simulink model "old_CascadePID_sim_v1"  (R2024b)
settings: Solver=ode4  StartTime=0.0  StopTime=30  FixedStep=0.05  RelTol=1e-3
values from neighbouring files (symbols this model uses):
  b_moment = 5.4e-6    (= 5.4e-06)    [CascadePID_matlab_client_v1.m]    (also in old_CascadePID_matlab_client_v1.m)
  k_thrust = 2.3e-3    (= 0.0023)    [CascadePID_matlab_client_v1.m]    (also in old_CascadePID_matlab_client_v1.m)
  l = 0.2051    [CascadePID_matlab_client_v1.m]    (also in old_CascadePID_matlab_client_v1.m)
libraries: slpidlib x9, simulink_extras x7
settings Model: Creator=Admin  LastModifiedBy=Admin

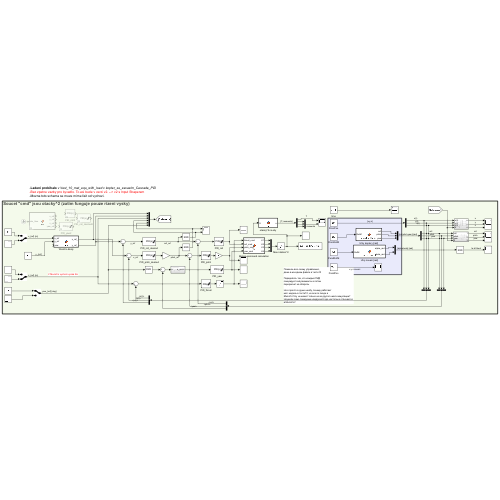
[thumbnail: Simulink's stored preview of the top-level diagram]
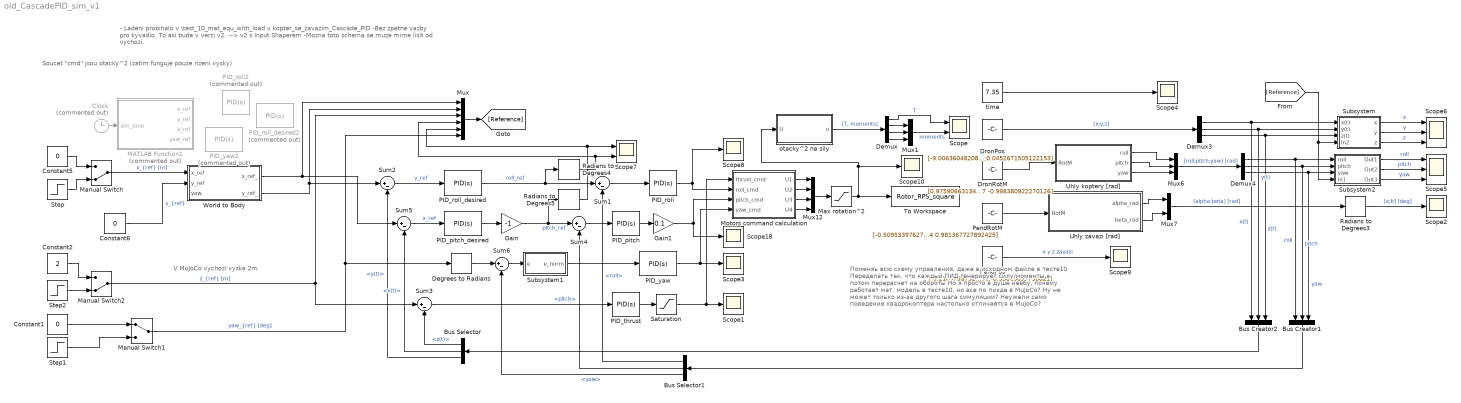
== system old_CascadePID_sim_v1 ==
  note: Поменяь всю схему управления,
      | даже в исходном файле в тесте10
      |
      | Переделать так, что каждый ПИД
      | генерирует силу/моменты а потом
      | перерасчет на обороты
      |
      | Но я просто в душе неебу, почему работает
      | мат. модель в тесте10, но все по пизде в
      | MuJoCo? Ну не может только из-за другого шага симуляции?
      | Неужели само поведение квадрокоптера настолько отличается
      | в MuJoCo?
  note: V MuJoCo vychozi vyska 2m
  note: - Ladeni probihalo v \test_10_mat_equ_with_load v kopter_se_zavazim_Cascade_PID
      | -Bez zpetne vazby pro kyvadlo. To asi bude v verzi v2. --> v2 s Input Shaperem
      | -Mozna toto schema se muze mirne lisit od vychozi.
  note: Soucet "cmd" jsou otacky^2 (zatim funguje pouze rizeni vysky)
  Bus Creator1 : BusCreator  Inputs=3
  Bus Creator2 : BusCreator  Inputs=3
  Bus Selector : BusSelector  OutputSignals=z(t),x(t),y(t)
  Bus Selector1 : BusSelector  OutputSignals=roll,pitch,yaw
  Clock : Clock  Commented=on
  Constant1 : Constant  Value=0
  Constant2 : Constant  Value=2
  Constant5 : Constant  Value=0
  Constant6 : Constant  Value=0
  Degrees to Radians : simulink_extras/Transformations/Degrees to Radians
  Demux : Demux
  Demux3 : Demux  Outputs=3
  Demux4 : Demux  Outputs=3
  DronPos : Constant  Value=[-9.00636048208464;0.341459514164713;0.0452671505122153]  SampleTime=-1
  DronRotM : Constant  Value=[0.975906631347119 0.216434408196844 -0.0276114802428831;0.214907774343092 -0.975367370953657 -0.0497306767081764;-0.0376947664752024 0.0425985754155727 -0.998380922270126]  SampleTime=-1
  Gain : Gain  Gain=-1
  Gain1 : Gain  Gain=0.1
  MATLAB Function1 : MATLAB Function  Commented=on  TreatAsAtomicUnit=on
  Manual Switch : ManualSwitch  CurrentSetting=0
  Manual Switch1 : ManualSwitch
  Manual Switch2 : ManualSwitch  CurrentSetting=0
  Max rotation^2 : Saturate  UpperLimit=4200  LowerLimit=0  LinearizeAsGain=off
  Motors command calculation : MATLAB Function  TreatAsAtomicUnit=on
  Mux : Mux  Inputs=6
  Mux1 : Mux  Inputs=3
  Mux12 : Mux
  Mux6 : Mux  Inputs=3
  Mux7 : Mux  Inputs=2
  PID_pitch : slpidlib/PID Controller  Controller=PID  Form=Parallel  TimeDomain=Continuous-time  UseExternalTs=off  SampleTime=-1  IntegratorMethod=Forward Euler  FilterMethod=Forward Euler  ControllerParametersSource=internal  P=218.455453578619  I=102.269436232904  UseKiTs=off  D=114.583796831467  UseExternalDerivativeSource=off  N=54.5397025421619  UseFilter=on  TunerSelectOption=Transfer Function Based (PID Tuner App)  InitialConditionSource=internal  InitialConditionForIntegrator=0  InitialConditionForFilter=0  DifferentiatorICPrevScaledInput=0  ExternalReset=none  TrackingMode=off  Kt=1  LimitOutput=on  SatLimitsSource=internal  UpperSaturationLimit=500  LowerSaturationLimit=-500  LinearizeAsGain=off  AntiWindupMode=clamping  Kb=1  LimitIntegrator=off  UpperIntegratorSaturationLimit=inf  LowerIntegratorSaturationLimit=-inf  POutMin=[]  POutMax=[]  IOutMin=[]  IOutMax=[]  DOutMin=[]  DOutMax=[]  NOutMin=[]  NOutMax=[]  SumOutMin=[]  SumOutMax=[]  SaturationOutMin=[]  SaturationOutMax=[]  PParamMin=[]  PParamMax=[]  IParamMin=[]  IParamMax=[]  DParamMin=[]  DParamMax=[]  NParamMin=[]  NParamMax=[]  KbParamMin=[]  KbParamMax=[]  KtParamMin=[]  KtParamMax=[]  KbOutMin=[]  KbOutMax=[]  KtOutMin=[]  KtOutMax=[]  IntegratorOutMin=[]  IntegratorOutMax=[]  FilterOutMin=[]  FilterOutMax=[]  SumI1OutMin=[]  SumI1OutMax=[]  SumI2OutMin=[]  SumI2OutMax=[]  SumI3OutMin=[]  SumI3OutMax=[]  SumI4OutMin=[]  SumI4OutMax=[]  SumDOutMin=[]  SumDOutMax=[]  DifferentiatorOutMin=[]  DifferentiatorOutMax=[]  FilterDiffOutCoefMin=[]  FilterDiffOutCoefMax=[]  ReciprocalOutMin=[]  ReciprocalOutMax=[]  SumDenOutMin=[]  SumDenOutMax=[]  SumNumOutMin=[]  SumNumOutMax=[]  DivideOutMin=[]  DivideOutMax=[]  UdiffTsProdOutMin=[]  UdiffTsProdOutMax=[]  NTsProdOutMin=[]  NTsProdOutMax=[]  UintegralTsProdOutMin=[]  UintegralTsProdOutMax=[]  UngainTsProdOutMin=[]  UngainTsProdOutMax=[]  ClampingZeroOutDataTypeStr=Inherit: Inherit via back propagation  ClampingZeroOutMin=[]  ClampingZeroOutMax=[]  FilterDenConstantOutDataTypeStr=Inherit: Inherit via back propagation  FilterDenConstantOutMin=[]  FilterDenConstantOutMax=[]  PCopyOutDataTypeStr=Inherit: Inherit via back propagation  PCopyOutMin=[]  PCopyOutMax=[]  NCopyOutDataTypeStr=Inherit: Inherit via back propagation  NCopyOutMin=[]  NCopyOutMax=[]  IntegratorContinuousStateAttributes=''  IntegratorStateMustResolveToSignalObject=off  IntegratorRTWStateStorageClass=Auto  FilterContinuousStateAttributes=''  FilterStateMustResolveToSignalObject=off  FilterRTWStateStorageClass=Auto  ParallelPVariant=InternalParameters  IdealPVariant=Disabled  IVariant=InternalParameters  DVariant=InternalParameters  IntegratorVariant=Continuous  SatVariant=Enabled  AWVariant=ContClampingParallel  PCopyVariant=Disabled  TRVariant=Disabled  FdbkBlocksVariant=Forward  IdealPFdbkVariant=Disabled  SatFdbkVariant=Disabled  DerivativeFilterVariant=ContFilter  NVariant=InternalParameters  NCopyVariant=Disabled  FilterICVariant=InternalICsFilter  IntegratorICVariant=InternalICs  ExternalResetVariant=Disabled  TRSumVariant=Passthrough  SumFdbkVariant=Disabled  SumVariant=Sum_PID  TsampFilterVariant=InternalTs  TsampNgainVariant=Passthrough  TsampIntegralVariant=Disabled_SignalSpec  ExternalSaturationOutDataTypeStr=Inherit: Same as second input  DerivativeSourceVariant=ErrorSignal  PreIntVariant=InternalPreInt
  PID_pitch_desired : slpidlib/PID Controller  Controller=PID  Form=Parallel  TimeDomain=Continuous-time  UseExternalTs=off  SampleTime=-1  IntegratorMethod=Forward Euler  FilterMethod=Forward Euler  ControllerParametersSource=internal  P=-0.0958604126455568  I=-0.00355407713511052  UseKiTs=off  D=-0.176236133491369  UseExternalDerivativeSource=off  N=18.7292151918558  UseFilter=on  TunerSelectOption=Transfer Function Based (PID Tuner App)  InitialConditionSource=internal  InitialConditionForIntegrator=0  InitialConditionForFilter=0  DifferentiatorICPrevScaledInput=0  ExternalReset=none  TrackingMode=off  Kt=1  LimitOutput=on  SatLimitsSource=internal  UpperSaturationLimit=45*pi/180  LowerSaturationLimit=-45*pi/180  LinearizeAsGain=on  AntiWindupMode=clamping  Kb=1  LimitIntegrator=off  UpperIntegratorSaturationLimit=inf  LowerIntegratorSaturationLimit=-inf  POutMin=[]  POutMax=[]  IOutMin=[]  IOutMax=[]  DOutMin=[]  DOutMax=[]  NOutMin=[]  NOutMax=[]  SumOutMin=[]  SumOutMax=[]  SaturationOutMin=[]  SaturationOutMax=[]  PParamMin=[]  PParamMax=[]  IParamMin=[]  IParamMax=[]  DParamMin=[]  DParamMax=[]  NParamMin=[]  NParamMax=[]  KbParamMin=[]  KbParamMax=[]  KtParamMin=[]  KtParamMax=[]  KbOutMin=[]  KbOutMax=[]  KtOutMin=[]  KtOutMax=[]  IntegratorOutMin=[]  IntegratorOutMax=[]  FilterOutMin=[]  FilterOutMax=[]  SumI1OutMin=[]  SumI1OutMax=[]  SumI2OutMin=[]  SumI2OutMax=[]  SumI3OutMin=[]  SumI3OutMax=[]  SumI4OutMin=[]  SumI4OutMax=[]  SumDOutMin=[]  SumDOutMax=[]  DifferentiatorOutMin=[]  DifferentiatorOutMax=[]  FilterDiffOutCoefMin=[]  FilterDiffOutCoefMax=[]  ReciprocalOutMin=[]  ReciprocalOutMax=[]  SumDenOutMin=[]  SumDenOutMax=[]  SumNumOutMin=[]  SumNumOutMax=[]  DivideOutMin=[]  DivideOutMax=[]  UdiffTsProdOutMin=[]  UdiffTsProdOutMax=[]  NTsProdOutMin=[]  NTsProdOutMax=[]  UintegralTsProdOutMin=[]  UintegralTsProdOutMax=[]  UngainTsProdOutMin=[]  UngainTsProdOutMax=[]  ClampingZeroOutDataTypeStr=Inherit: Inherit via back propagation  ClampingZeroOutMin=[]  ClampingZeroOutMax=[]  FilterDenConstantOutDataTypeStr=Inherit: Inherit via back propagation  FilterDenConstantOutMin=[]  FilterDenConstantOutMax=[]  PCopyOutDataTypeStr=Inherit: Inherit via back propagation  PCopyOutMin=[]  PCopyOutMax=[]  NCopyOutDataTypeStr=Inherit: Inherit via back propagation  NCopyOutMin=[]  NCopyOutMax=[]  IntegratorContinuousStateAttributes=''  IntegratorStateMustResolveToSignalObject=off  IntegratorRTWStateStorageClass=Auto  FilterContinuousStateAttributes=''  FilterStateMustResolveToSignalObject=off  FilterRTWStateStorageClass=Auto  ParallelPVariant=InternalParameters  IdealPVariant=Disabled  IVariant=InternalParameters  DVariant=InternalParameters  IntegratorVariant=Continuous  SatVariant=Enabled  AWVariant=ContClampingParallel  PCopyVariant=Disabled  TRVariant=Disabled  FdbkBlocksVariant=Forward  IdealPFdbkVariant=Disabled  SatFdbkVariant=Disabled  DerivativeFilterVariant=ContFilter  NVariant=InternalParameters  NCopyVariant=Disabled  FilterICVariant=InternalICsFilter  IntegratorICVariant=InternalICs  ExternalResetVariant=Disabled  TRSumVariant=Passthrough  SumFdbkVariant=Disabled  SumVariant=Sum_PID  TsampFilterVariant=InternalTs  TsampNgainVariant=Passthrough  TsampIntegralVariant=Disabled_SignalSpec  ExternalSaturationOutDataTypeStr=Inherit: Same as second input  DerivativeSourceVariant=ErrorSignal  PreIntVariant=InternalPreInt
  PID_roll : slpidlib/PID Controller  Controller=PID  Form=Parallel  TimeDomain=Continuous-time  UseExternalTs=off  SampleTime=-1  IntegratorMethod=Forward Euler  FilterMethod=Forward Euler  ControllerParametersSource=internal  P=218.455453578619  I=102.269436232904  UseKiTs=off  D=114.583796831467  UseExternalDerivativeSource=off  N=54.5397025421619  UseFilter=on  TunerSelectOption=Transfer Function Based (PID Tuner App)  InitialConditionSource=internal  InitialConditionForIntegrator=0  InitialConditionForFilter=0  DifferentiatorICPrevScaledInput=0  ExternalReset=none  TrackingMode=off  Kt=1  LimitOutput=on  SatLimitsSource=internal  UpperSaturationLimit=500  LowerSaturationLimit=-500  LinearizeAsGain=off  AntiWindupMode=clamping  Kb=1  LimitIntegrator=off  UpperIntegratorSaturationLimit=inf  LowerIntegratorSaturationLimit=-inf  POutMin=[]  POutMax=[]  IOutMin=[]  IOutMax=[]  DOutMin=[]  DOutMax=[]  NOutMin=[]  NOutMax=[]  SumOutMin=[]  SumOutMax=[]  SaturationOutMin=[]  SaturationOutMax=[]  PParamMin=[]  PParamMax=[]  IParamMin=[]  IParamMax=[]  DParamMin=[]  DParamMax=[]  NParamMin=[]  NParamMax=[]  KbParamMin=[]  KbParamMax=[]  KtParamMin=[]  KtParamMax=[]  KbOutMin=[]  KbOutMax=[]  KtOutMin=[]  KtOutMax=[]  IntegratorOutMin=[]  IntegratorOutMax=[]  FilterOutMin=[]  FilterOutMax=[]  SumI1OutMin=[]  SumI1OutMax=[]  SumI2OutMin=[]  SumI2OutMax=[]  SumI3OutMin=[]  SumI3OutMax=[]  SumI4OutMin=[]  SumI4OutMax=[]  SumDOutMin=[]  SumDOutMax=[]  DifferentiatorOutMin=[]  DifferentiatorOutMax=[]  FilterDiffOutCoefMin=[]  FilterDiffOutCoefMax=[]  ReciprocalOutMin=[]  ReciprocalOutMax=[]  SumDenOutMin=[]  SumDenOutMax=[]  SumNumOutMin=[]  SumNumOutMax=[]  DivideOutMin=[]  DivideOutMax=[]  UdiffTsProdOutMin=[]  UdiffTsProdOutMax=[]  NTsProdOutMin=[]  NTsProdOutMax=[]  UintegralTsProdOutMin=[]  UintegralTsProdOutMax=[]  UngainTsProdOutMin=[]  UngainTsProdOutMax=[]  ClampingZeroOutDataTypeStr=Inherit: Inherit via back propagation  ClampingZeroOutMin=[]  ClampingZeroOutMax=[]  FilterDenConstantOutDataTypeStr=Inherit: Inherit via back propagation  FilterDenConstantOutMin=[]  FilterDenConstantOutMax=[]  PCopyOutDataTypeStr=Inherit: Inherit via back propagation  PCopyOutMin=[]  PCopyOutMax=[]  NCopyOutDataTypeStr=Inherit: Inherit via back propagation  NCopyOutMin=[]  NCopyOutMax=[]  IntegratorContinuousStateAttributes=''  IntegratorStateMustResolveToSignalObject=off  IntegratorRTWStateStorageClass=Auto  FilterContinuousStateAttributes=''  FilterStateMustResolveToSignalObject=off  FilterRTWStateStorageClass=Auto  ParallelPVariant=InternalParameters  IdealPVariant=Disabled  IVariant=InternalParameters  DVariant=InternalParameters  IntegratorVariant=Continuous  SatVariant=Enabled  AWVariant=ContClampingParallel  PCopyVariant=Disabled  TRVariant=Disabled  FdbkBlocksVariant=Forward  IdealPFdbkVariant=Disabled  SatFdbkVariant=Disabled  DerivativeFilterVariant=ContFilter  NVariant=InternalParameters  NCopyVariant=Disabled  FilterICVariant=InternalICsFilter  IntegratorICVariant=InternalICs  ExternalResetVariant=Disabled  TRSumVariant=Passthrough  SumFdbkVariant=Disabled  SumVariant=Sum_PID  TsampFilterVariant=InternalTs  TsampNgainVariant=Passthrough  TsampIntegralVariant=Disabled_SignalSpec  ExternalSaturationOutDataTypeStr=Inherit: Same as second input  DerivativeSourceVariant=ErrorSignal  PreIntVariant=InternalPreInt
  PID_roll2 : slpidlib/PID Controller  Commented=on  Controller=PID  Form=Parallel  TimeDomain=Continuous-time  UseExternalTs=off  SampleTime=-1  IntegratorMethod=Forward Euler  FilterMethod=Forward Euler  ControllerParametersSource=internal  P=42.2441725722026  I=1.18935330465342  UseKiTs=off  D=40.9229138980428  UseExternalDerivativeSource=off  N=3.31131121482591  UseFilter=on  TunerSelectOption=Transfer Function Based (PID Tuner App)  InitialConditionSource=internal  InitialConditionForIntegrator=0  InitialConditionForFilter=0  DifferentiatorICPrevScaledInput=0  ExternalReset=none  TrackingMode=off  Kt=1  LimitOutput=off  SatLimitsSource=internal  UpperSaturationLimit=15  LowerSaturationLimit=-15  LinearizeAsGain=on  AntiWindupMode=none  Kb=1  LimitIntegrator=off  UpperIntegratorSaturationLimit=inf  LowerIntegratorSaturationLimit=-inf  POutMin=[]  POutMax=[]  IOutMin=[]  IOutMax=[]  DOutMin=[]  DOutMax=[]  NOutMin=[]  NOutMax=[]  SumOutMin=[]  SumOutMax=[]  SaturationOutMin=[]  SaturationOutMax=[]  PParamMin=[]  PParamMax=[]  IParamMin=[]  IParamMax=[]  DParamMin=[]  DParamMax=[]  NParamMin=[]  NParamMax=[]  KbParamMin=[]  KbParamMax=[]  KtParamMin=[]  KtParamMax=[]  KbOutMin=[]  KbOutMax=[]  KtOutMin=[]  KtOutMax=[]  IntegratorOutMin=[]  IntegratorOutMax=[]  FilterOutMin=[]  FilterOutMax=[]  SumI1OutMin=[]  SumI1OutMax=[]  SumI2OutMin=[]  SumI2OutMax=[]  SumI3OutMin=[]  SumI3OutMax=[]  SumI4OutMin=[]  SumI4OutMax=[]  SumDOutMin=[]  SumDOutMax=[]  DifferentiatorOutMin=[]  DifferentiatorOutMax=[]  FilterDiffOutCoefMin=[]  FilterDiffOutCoefMax=[]  ReciprocalOutMin=[]  ReciprocalOutMax=[]  SumDenOutMin=[]  SumDenOutMax=[]  SumNumOutMin=[]  SumNumOutMax=[]  DivideOutMin=[]  DivideOutMax=[]  UdiffTsProdOutMin=[]  UdiffTsProdOutMax=[]  NTsProdOutMin=[]  NTsProdOutMax=[]  UintegralTsProdOutMin=[]  UintegralTsProdOutMax=[]  UngainTsProdOutMin=[]  UngainTsProdOutMax=[]  ClampingZeroOutDataTypeStr=Inherit: Inherit via back propagation  ClampingZeroOutMin=[]  ClampingZeroOutMax=[]  FilterDenConstantOutDataTypeStr=Inherit: Inherit via back propagation  FilterDenConstantOutMin=[]  FilterDenConstantOutMax=[]  PCopyOutDataTypeStr=Inherit: Inherit via back propagation  PCopyOutMin=[]  PCopyOutMax=[]  NCopyOutDataTypeStr=Inherit: Inherit via back propagation  NCopyOutMin=[]  NCopyOutMax=[]  IntegratorContinuousStateAttributes=''  IntegratorStateMustResolveToSignalObject=off  IntegratorRTWStateStorageClass=Auto  FilterContinuousStateAttributes=''  FilterStateMustResolveToSignalObject=off  FilterRTWStateStorageClass=Auto  ParallelPVariant=InternalParameters  IdealPVariant=Disabled  IVariant=InternalParameters  DVariant=InternalParameters  IntegratorVariant=Continuous  SatVariant=Disabled  AWVariant=Passthrough  PCopyVariant=Disabled  TRVariant=Disabled  FdbkBlocksVariant=Forward  IdealPFdbkVariant=Disabled  SatFdbkVariant=Disabled  DerivativeFilterVariant=ContFilter  NVariant=InternalParameters  NCopyVariant=Disabled  FilterICVariant=InternalICsFilter  IntegratorICVariant=InternalICs  ExternalResetVariant=Disabled  TRSumVariant=Passthrough  SumFdbkVariant=Disabled  SumVariant=Sum_PID  TsampFilterVariant=InternalTs  TsampNgainVariant=Passthrough  TsampIntegralVariant=Disabled_SignalSpec  ExternalSaturationOutDataTypeStr=Inherit: Same as second input  DerivativeSourceVariant=ErrorSignal  PreIntVariant=InternalPreInt
  PID_roll_desired : slpidlib/PID Controller  Controller=PID  Form=Parallel  TimeDomain=Continuous-time  UseExternalTs=off  SampleTime=-1  IntegratorMethod=Forward Euler  FilterMethod=Forward Euler  ControllerParametersSource=internal  P=-0.0958604126455568  I=-0.00355407713511052  UseKiTs=off  D=-0.176236133491369  UseExternalDerivativeSource=off  N=18.7292151918558  UseFilter=on  TunerSelectOption=Transfer Function Based (PID Tuner App)  InitialConditionSource=internal  InitialConditionForIntegrator=0  InitialConditionForFilter=0  DifferentiatorICPrevScaledInput=0  ExternalReset=none  TrackingMode=off  Kt=1  LimitOutput=on  SatLimitsSource=internal  UpperSaturationLimit=45*pi/180  LowerSaturationLimit=-45*pi/180  LinearizeAsGain=on  AntiWindupMode=clamping  Kb=1  LimitIntegrator=off  UpperIntegratorSaturationLimit=inf  LowerIntegratorSaturationLimit=-inf  POutMin=[]  POutMax=[]  IOutMin=[]  IOutMax=[]  DOutMin=[]  DOutMax=[]  NOutMin=[]  NOutMax=[]  SumOutMin=[]  SumOutMax=[]  SaturationOutMin=[]  SaturationOutMax=[]  PParamMin=[]  PParamMax=[]  IParamMin=[]  IParamMax=[]  DParamMin=[]  DParamMax=[]  NParamMin=[]  NParamMax=[]  KbParamMin=[]  KbParamMax=[]  KtParamMin=[]  KtParamMax=[]  KbOutMin=[]  KbOutMax=[]  KtOutMin=[]  KtOutMax=[]  IntegratorOutMin=[]  IntegratorOutMax=[]  FilterOutMin=[]  FilterOutMax=[]  SumI1OutMin=[]  SumI1OutMax=[]  SumI2OutMin=[]  SumI2OutMax=[]  SumI3OutMin=[]  SumI3OutMax=[]  SumI4OutMin=[]  SumI4OutMax=[]  SumDOutMin=[]  SumDOutMax=[]  DifferentiatorOutMin=[]  DifferentiatorOutMax=[]  FilterDiffOutCoefMin=[]  FilterDiffOutCoefMax=[]  ReciprocalOutMin=[]  ReciprocalOutMax=[]  SumDenOutMin=[]  SumDenOutMax=[]  SumNumOutMin=[]  SumNumOutMax=[]  DivideOutMin=[]  DivideOutMax=[]  UdiffTsProdOutMin=[]  UdiffTsProdOutMax=[]  NTsProdOutMin=[]  NTsProdOutMax=[]  UintegralTsProdOutMin=[]  UintegralTsProdOutMax=[]  UngainTsProdOutMin=[]  UngainTsProdOutMax=[]  ClampingZeroOutDataTypeStr=Inherit: Inherit via back propagation  ClampingZeroOutMin=[]  ClampingZeroOutMax=[]  FilterDenConstantOutDataTypeStr=Inherit: Inherit via back propagation  FilterDenConstantOutMin=[]  FilterDenConstantOutMax=[]  PCopyOutDataTypeStr=Inherit: Inherit via back propagation  PCopyOutMin=[]  PCopyOutMax=[]  NCopyOutDataTypeStr=Inherit: Inherit via back propagation  NCopyOutMin=[]  NCopyOutMax=[]  IntegratorContinuousStateAttributes=''  IntegratorStateMustResolveToSignalObject=off  IntegratorRTWStateStorageClass=Auto  FilterContinuousStateAttributes=''  FilterStateMustResolveToSignalObject=off  FilterRTWStateStorageClass=Auto  ParallelPVariant=InternalParameters  IdealPVariant=Disabled  IVariant=InternalParameters  DVariant=InternalParameters  IntegratorVariant=Continuous  SatVariant=Enabled  AWVariant=ContClampingParallel  PCopyVariant=Disabled  TRVariant=Disabled  FdbkBlocksVariant=Forward  IdealPFdbkVariant=Disabled  SatFdbkVariant=Disabled  DerivativeFilterVariant=ContFilter  NVariant=InternalParameters  NCopyVariant=Disabled  FilterICVariant=InternalICsFilter  IntegratorICVariant=InternalICs  ExternalResetVariant=Disabled  TRSumVariant=Passthrough  SumFdbkVariant=Disabled  SumVariant=Sum_PID  TsampFilterVariant=InternalTs  TsampNgainVariant=Passthrough  TsampIntegralVariant=Disabled_SignalSpec  ExternalSaturationOutDataTypeStr=Inherit: Same as second input  DerivativeSourceVariant=ErrorSignal  PreIntVariant=InternalPreInt
  PID_roll_desired2 : slpidlib/PID Controller  Commented=on  Controller=PID  Form=Parallel  TimeDomain=Continuous-time  UseExternalTs=off  SampleTime=-1  IntegratorMethod=Forward Euler  FilterMethod=Forward Euler  ControllerParametersSource=internal  P=-0.0199563159997824  I=-0.00105353798256793  UseKiTs=off  D=-0.0719369452769512  UseExternalDerivativeSource=off  N=85.0622233198974  UseFilter=on  TunerSelectOption=Transfer Function Based (PID Tuner App)  InitialConditionSource=internal  InitialConditionForIntegrator=0  InitialConditionForFilter=0  DifferentiatorICPrevScaledInput=0  ExternalReset=none  TrackingMode=off  Kt=1  LimitOutput=on  SatLimitsSource=internal  UpperSaturationLimit=45*pi/180  LowerSaturationLimit=-45*pi/180  LinearizeAsGain=on  AntiWindupMode=clamping  Kb=1  LimitIntegrator=off  UpperIntegratorSaturationLimit=inf  LowerIntegratorSaturationLimit=-inf  POutMin=[]  POutMax=[]  IOutMin=[]  IOutMax=[]  DOutMin=[]  DOutMax=[]  NOutMin=[]  NOutMax=[]  SumOutMin=[]  SumOutMax=[]  SaturationOutMin=[]  SaturationOutMax=[]  PParamMin=[]  PParamMax=[]  IParamMin=[]  IParamMax=[]  DParamMin=[]  DParamMax=[]  NParamMin=[]  NParamMax=[]  KbParamMin=[]  KbParamMax=[]  KtParamMin=[]  KtParamMax=[]  KbOutMin=[]  KbOutMax=[]  KtOutMin=[]  KtOutMax=[]  IntegratorOutMin=[]  IntegratorOutMax=[]  FilterOutMin=[]  FilterOutMax=[]  SumI1OutMin=[]  SumI1OutMax=[]  SumI2OutMin=[]  SumI2OutMax=[]  SumI3OutMin=[]  SumI3OutMax=[]  SumI4OutMin=[]  SumI4OutMax=[]  SumDOutMin=[]  SumDOutMax=[]  DifferentiatorOutMin=[]  DifferentiatorOutMax=[]  FilterDiffOutCoefMin=[]  FilterDiffOutCoefMax=[]  ReciprocalOutMin=[]  ReciprocalOutMax=[]  SumDenOutMin=[]  SumDenOutMax=[]  SumNumOutMin=[]  SumNumOutMax=[]  DivideOutMin=[]  DivideOutMax=[]  UdiffTsProdOutMin=[]  UdiffTsProdOutMax=[]  NTsProdOutMin=[]  NTsProdOutMax=[]  UintegralTsProdOutMin=[]  UintegralTsProdOutMax=[]  UngainTsProdOutMin=[]  UngainTsProdOutMax=[]  ClampingZeroOutDataTypeStr=Inherit: Inherit via back propagation  ClampingZeroOutMin=[]  ClampingZeroOutMax=[]  FilterDenConstantOutDataTypeStr=Inherit: Inherit via back propagation  FilterDenConstantOutMin=[]  FilterDenConstantOutMax=[]  PCopyOutDataTypeStr=Inherit: Inherit via back propagation  PCopyOutMin=[]  PCopyOutMax=[]  NCopyOutDataTypeStr=Inherit: Inherit via back propagation  NCopyOutMin=[]  NCopyOutMax=[]  IntegratorContinuousStateAttributes=''  IntegratorStateMustResolveToSignalObject=off  IntegratorRTWStateStorageClass=Auto  FilterContinuousStateAttributes=''  FilterStateMustResolveToSignalObject=off  FilterRTWStateStorageClass=Auto  ParallelPVariant=InternalParameters  IdealPVariant=Disabled  IVariant=InternalParameters  DVariant=InternalParameters  IntegratorVariant=Continuous  SatVariant=Enabled  AWVariant=ContClampingParallel  PCopyVariant=Disabled  TRVariant=Disabled  FdbkBlocksVariant=Forward  IdealPFdbkVariant=Disabled  SatFdbkVariant=Disabled  DerivativeFilterVariant=ContFilter  NVariant=InternalParameters  NCopyVariant=Disabled  FilterICVariant=InternalICsFilter  IntegratorICVariant=InternalICs  ExternalResetVariant=Disabled  TRSumVariant=Passthrough  SumFdbkVariant=Disabled  SumVariant=Sum_PID  TsampFilterVariant=InternalTs  TsampNgainVariant=Passthrough  TsampIntegralVariant=Disabled_SignalSpec  ExternalSaturationOutDataTypeStr=Inherit: Same as second input  DerivativeSourceVariant=ErrorSignal  PreIntVariant=InternalPreInt
  PID_thrust : slpidlib/PID Controller  Controller=PID  Form=Parallel  TimeDomain=Continuous-time  UseExternalTs=off  SampleTime=-1  IntegratorMethod=Forward Euler  FilterMethod=Forward Euler  ControllerParametersSource=internal  P=605.475858467149  I=89.6354498687062  UseKiTs=off  D=1004.2854008956  UseExternalDerivativeSource=off  N=17.2469682941307  UseFilter=on  TunerSelectOption=Transfer Function Based (PID Tuner App)  InitialConditionSource=internal  InitialConditionForIntegrator=3198.9  InitialConditionForFilter=0  DifferentiatorICPrevScaledInput=0  ExternalReset=none  TrackingMode=off  Kt=1  LimitOutput=on  SatLimitsSource=internal  UpperSaturationLimit=4200  LowerSaturationLimit=0  LinearizeAsGain=off  AntiWindupMode=clamping  Kb=1  LimitIntegrator=off  UpperIntegratorSaturationLimit=inf  LowerIntegratorSaturationLimit=-inf  POutMin=[]  POutMax=[]  IOutMin=[]  IOutMax=[]  DOutMin=[]  DOutMax=[]  NOutMin=[]  NOutMax=[]  SumOutMin=[]  SumOutMax=[]  SaturationOutMin=[]  SaturationOutMax=[]  PParamMin=[]  PParamMax=[]  IParamMin=[]  IParamMax=[]  DParamMin=[]  DParamMax=[]  NParamMin=[]  NParamMax=[]  KbParamMin=[]  KbParamMax=[]  KtParamMin=[]  KtParamMax=[]  KbOutMin=[]  KbOutMax=[]  KtOutMin=[]  KtOutMax=[]  IntegratorOutMin=[]  IntegratorOutMax=[]  FilterOutMin=[]  FilterOutMax=[]  SumI1OutMin=[]  SumI1OutMax=[]  SumI2OutMin=[]  SumI2OutMax=[]  SumI3OutMin=[]  SumI3OutMax=[]  SumI4OutMin=[]  SumI4OutMax=[]  SumDOutMin=[]  SumDOutMax=[]  DifferentiatorOutMin=[]  DifferentiatorOutMax=[]  FilterDiffOutCoefMin=[]  FilterDiffOutCoefMax=[]  ReciprocalOutMin=[]  ReciprocalOutMax=[]  SumDenOutMin=[]  SumDenOutMax=[]  SumNumOutMin=[]  SumNumOutMax=[]  DivideOutMin=[]  DivideOutMax=[]  UdiffTsProdOutMin=[]  UdiffTsProdOutMax=[]  NTsProdOutMin=[]  NTsProdOutMax=[]  UintegralTsProdOutMin=[]  UintegralTsProdOutMax=[]  UngainTsProdOutMin=[]  UngainTsProdOutMax=[]  ClampingZeroOutDataTypeStr=Inherit: Inherit via back propagation  ClampingZeroOutMin=[]  ClampingZeroOutMax=[]  FilterDenConstantOutDataTypeStr=Inherit: Inherit via back propagation  FilterDenConstantOutMin=[]  FilterDenConstantOutMax=[]  PCopyOutDataTypeStr=Inherit: Inherit via back propagation  PCopyOutMin=[]  PCopyOutMax=[]  NCopyOutDataTypeStr=Inherit: Inherit via back propagation  NCopyOutMin=[]  NCopyOutMax=[]  IntegratorContinuousStateAttributes=''  IntegratorStateMustResolveToSignalObject=off  IntegratorRTWStateStorageClass=Auto  FilterContinuousStateAttributes=''  FilterStateMustResolveToSignalObject=off  FilterRTWStateStorageClass=Auto  ParallelPVariant=InternalParameters  IdealPVariant=Disabled  IVariant=InternalParameters  DVariant=InternalParameters  IntegratorVariant=Continuous  SatVariant=Enabled  AWVariant=ContClampingParallel  PCopyVariant=Disabled  TRVariant=Disabled  FdbkBlocksVariant=Forward  IdealPFdbkVariant=Disabled  SatFdbkVariant=Disabled  DerivativeFilterVariant=ContFilter  NVariant=InternalParameters  NCopyVariant=Disabled  FilterICVariant=InternalICsFilter  IntegratorICVariant=InternalICs  ExternalResetVariant=Disabled  TRSumVariant=Passthrough  SumFdbkVariant=Disabled  SumVariant=Sum_PID  TsampFilterVariant=InternalTs  TsampNgainVariant=Passthrough  TsampIntegralVariant=Disabled_SignalSpec  ExternalSaturationOutDataTypeStr=Inherit: Same as second input  DerivativeSourceVariant=ErrorSignal  PreIntVariant=InternalPreInt
  PID_yaw : slpidlib/PID Controller  Controller=PID  Form=Parallel  TimeDomain=Continuous-time  UseExternalTs=off  SampleTime=-1  IntegratorMethod=Forward Euler  FilterMethod=Forward Euler  ControllerParametersSource=internal  P=1765.09036919174  I=180.779806074397  UseKiTs=off  D=4231.82074465776  UseExternalDerivativeSource=off  N=11.9319868203366  UseFilter=on  TunerSelectOption=Transfer Function Based (PID Tuner App)  InitialConditionSource=internal  InitialConditionForIntegrator=0  InitialConditionForFilter=0  DifferentiatorICPrevScaledInput=0  ExternalReset=none  TrackingMode=off  Kt=1  LimitOutput=on  SatLimitsSource=internal  UpperSaturationLimit=700  LowerSaturationLimit=-700  LinearizeAsGain=off  AntiWindupMode=clamping  Kb=1  LimitIntegrator=off  UpperIntegratorSaturationLimit=inf  LowerIntegratorSaturationLimit=-inf  POutMin=[]  POutMax=[]  IOutMin=[]  IOutMax=[]  DOutMin=[]  DOutMax=[]  NOutMin=[]  NOutMax=[]  SumOutMin=[]  SumOutMax=[]  SaturationOutMin=[]  SaturationOutMax=[]  PParamMin=[]  PParamMax=[]  IParamMin=[]  IParamMax=[]  DParamMin=[]  DParamMax=[]  NParamMin=[]  NParamMax=[]  KbParamMin=[]  KbParamMax=[]  KtParamMin=[]  KtParamMax=[]  KbOutMin=[]  KbOutMax=[]  KtOutMin=[]  KtOutMax=[]  IntegratorOutMin=[]  IntegratorOutMax=[]  FilterOutMin=[]  FilterOutMax=[]  SumI1OutMin=[]  SumI1OutMax=[]  SumI2OutMin=[]  SumI2OutMax=[]  SumI3OutMin=[]  SumI3OutMax=[]  SumI4OutMin=[]  SumI4OutMax=[]  SumDOutMin=[]  SumDOutMax=[]  DifferentiatorOutMin=[]  DifferentiatorOutMax=[]  FilterDiffOutCoefMin=[]  FilterDiffOutCoefMax=[]  ReciprocalOutMin=[]  ReciprocalOutMax=[]  SumDenOutMin=[]  SumDenOutMax=[]  SumNumOutMin=[]  SumNumOutMax=[]  DivideOutMin=[]  DivideOutMax=[]  UdiffTsProdOutMin=[]  UdiffTsProdOutMax=[]  NTsProdOutMin=[]  NTsProdOutMax=[]  UintegralTsProdOutMin=[]  UintegralTsProdOutMax=[]  UngainTsProdOutMin=[]  UngainTsProdOutMax=[]  ClampingZeroOutDataTypeStr=Inherit: Inherit via back propagation  ClampingZeroOutMin=[]  ClampingZeroOutMax=[]  FilterDenConstantOutDataTypeStr=Inherit: Inherit via back propagation  FilterDenConstantOutMin=[]  FilterDenConstantOutMax=[]  PCopyOutDataTypeStr=Inherit: Inherit via back propagation  PCopyOutMin=[]  PCopyOutMax=[]  NCopyOutDataTypeStr=Inherit: Inherit via back propagation  NCopyOutMin=[]  NCopyOutMax=[]  IntegratorContinuousStateAttributes=''  IntegratorStateMustResolveToSignalObject=off  IntegratorRTWStateStorageClass=Auto  FilterContinuousStateAttributes=''  FilterStateMustResolveToSignalObject=off  FilterRTWStateStorageClass=Auto  ParallelPVariant=InternalParameters  IdealPVariant=Disabled  IVariant=InternalParameters  DVariant=InternalParameters  IntegratorVariant=Continuous  SatVariant=Enabled  AWVariant=ContClampingParallel  PCopyVariant=Disabled  TRVariant=Disabled  FdbkBlocksVariant=Forward  IdealPFdbkVariant=Disabled  SatFdbkVariant=Disabled  DerivativeFilterVariant=ContFilter  NVariant=InternalParameters  NCopyVariant=Disabled  FilterICVariant=InternalICsFilter  IntegratorICVariant=InternalICs  ExternalResetVariant=Disabled  TRSumVariant=Passthrough  SumFdbkVariant=Disabled  SumVariant=Sum_PID  TsampFilterVariant=InternalTs  TsampNgainVariant=Passthrough  TsampIntegralVariant=Disabled_SignalSpec  ExternalSaturationOutDataTypeStr=Inherit: Same as second input  DerivativeSourceVariant=ErrorSignal  PreIntVariant=InternalPreInt
  PID_yaw2 : slpidlib/PID Controller  Commented=on  Controller=PID  Form=Parallel  TimeDomain=Continuous-time  UseExternalTs=off  SampleTime=-1  IntegratorMethod=Forward Euler  FilterMethod=Forward Euler  ControllerParametersSource=internal  P=1415.34348585472  I=118.509886072305  UseKiTs=off  D=4115.24841503536  UseExternalDerivativeSource=off  N=238.770606857548  UseFilter=on  TunerSelectOption=Transfer Function Based (PID Tuner App)  InitialConditionSource=internal  InitialConditionForIntegrator=0  InitialConditionForFilter=0  DifferentiatorICPrevScaledInput=0  ExternalReset=none  TrackingMode=off  Kt=1  LimitOutput=on  SatLimitsSource=internal  UpperSaturationLimit=1  LowerSaturationLimit=-1  LinearizeAsGain=off  AntiWindupMode=back-calculation  Kb=1  LimitIntegrator=off  UpperIntegratorSaturationLimit=inf  LowerIntegratorSaturationLimit=-inf  POutMin=[]  POutMax=[]  IOutMin=[]  IOutMax=[]  DOutMin=[]  DOutMax=[]  NOutMin=[]  NOutMax=[]  SumOutMin=[]  SumOutMax=[]  SaturationOutMin=[]  SaturationOutMax=[]  PParamMin=[]  PParamMax=[]  IParamMin=[]  IParamMax=[]  DParamMin=[]  DParamMax=[]  NParamMin=[]  NParamMax=[]  KbParamMin=[]  KbParamMax=[]  KtParamMin=[]  KtParamMax=[]  KbOutMin=[]  KbOutMax=[]  KtOutMin=[]  KtOutMax=[]  IntegratorOutMin=[]  IntegratorOutMax=[]  FilterOutMin=[]  FilterOutMax=[]  SumI1OutMin=[]  SumI1OutMax=[]  SumI2OutMin=[]  SumI2OutMax=[]  SumI3OutMin=[]  SumI3OutMax=[]  SumI4OutMin=[]  SumI4OutMax=[]  SumDOutMin=[]  SumDOutMax=[]  DifferentiatorOutMin=[]  DifferentiatorOutMax=[]  FilterDiffOutCoefMin=[]  FilterDiffOutCoefMax=[]  ReciprocalOutMin=[]  ReciprocalOutMax=[]  SumDenOutMin=[]  SumDenOutMax=[]  SumNumOutMin=[]  SumNumOutMax=[]  DivideOutMin=[]  DivideOutMax=[]  UdiffTsProdOutMin=[]  UdiffTsProdOutMax=[]  NTsProdOutMin=[]  NTsProdOutMax=[]  UintegralTsProdOutMin=[]  UintegralTsProdOutMax=[]  UngainTsProdOutMin=[]  UngainTsProdOutMax=[]  ClampingZeroOutDataTypeStr=Inherit: Inherit via back propagation  ClampingZeroOutMin=[]  ClampingZeroOutMax=[]  FilterDenConstantOutDataTypeStr=Inherit: Inherit via back propagation  FilterDenConstantOutMin=[]  FilterDenConstantOutMax=[]  PCopyOutDataTypeStr=Inherit: Inherit via back propagation  PCopyOutMin=[]  PCopyOutMax=[]  NCopyOutDataTypeStr=Inherit: Inherit via back propagation  NCopyOutMin=[]  NCopyOutMax=[]  IntegratorContinuousStateAttributes=''  IntegratorStateMustResolveToSignalObject=off  IntegratorRTWStateStorageClass=Auto  FilterContinuousStateAttributes=''  FilterStateMustResolveToSignalObject=off  FilterRTWStateStorageClass=Auto  ParallelPVariant=InternalParameters  IdealPVariant=Disabled  IVariant=InternalParameters  DVariant=InternalParameters  IntegratorVariant=Continuous  SatVariant=Enabled  AWVariant=BackCalculation  PCopyVariant=Disabled  TRVariant=Disabled  FdbkBlocksVariant=Forward  IdealPFdbkVariant=Disabled  SatFdbkVariant=Disabled  DerivativeFilterVariant=ContFilter  NVariant=InternalParameters  NCopyVariant=Disabled  FilterICVariant=InternalICsFilter  IntegratorICVariant=InternalICs  ExternalResetVariant=Disabled  TRSumVariant=Passthrough  SumFdbkVariant=Disabled  SumVariant=Sum_PID  TsampFilterVariant=InternalTs  TsampNgainVariant=Passthrough  TsampIntegralVariant=Disabled_SignalSpec  ExternalSaturationOutDataTypeStr=Inherit: Same as second input  DerivativeSourceVariant=ErrorSignal  PreIntVariant=InternalPreInt
  PendPos : Constant  Value=[-9.11857987523727;0.497421658455291;-0.93610057738021]  SampleTime=-1
  PendRotM : Constant  Value=[-0.509533976275694 -0.853101362571375 0.112219393152631;0.838852119791314 -0.521539002060156 -0.155962144290578;0.191578308120465 0.0146674642989174 0.981367727892425]  SampleTime=-1
  Radians to Degrees3 : simulink_extras/Transformations/Radians to Degrees
  Radians to Degrees4 : simulink_extras/Transformations/Radians to Degrees
  Radians to Degrees5 : simulink_extras/Transformations/Radians to Degrees
  Saturation : Saturate  UpperLimit=4200  LowerLimit=0
  Scope : Scope  NumInputPorts=2
  Scope{1..4,8..10,18} (8 alike) : Scope
  Scope5 : Scope  NumInputPorts=3
  Scope6 : Scope  NumInputPorts=3
  Scope7 : Scope  NumInputPorts=2
  Step : Step  Time=2  SampleTime=0
  Step1 : Step  Time=2  After=10  SampleTime=0
  Step2 : Step  Time=2  Before=2  After=3  SampleTime=0
  Subsystem : Subsystem
  Subsystem1 : Subsystem
  Subsystem2 : Subsystem
  Sum{1..6} (6 alike) : Sum  Inputs=|+-
  To Workspace : ToWorkspace  VariableName=Rotor_RPS_square  SampleTime=-1
  Uhly koptery [rad] : MATLAB Function  TreatAsAtomicUnit=on
  Uhly zavazi [rad] : MATLAB Function  TreatAsAtomicUnit=on
  World to Body : MATLAB Function  TreatAsAtomicUnit=on
  otacky^2 na sily : MATLAB Function  TreatAsAtomicUnit=on
  time : Constant  Value=7.35  SampleTime=-1
  wires:
  Sum2/1 -> PID_roll_desired/1  "y_ref"
  Bus Selector/3 -> Sum2/2  "<y(t)>"
  PID_yaw/1 -> Motors command calculation/4(yaw_cmd), Scope3/1
  Demux3/1 -> Subsystem/1(x(t)), Bus Creator2/1  "x(t)"
  Sum3/1 -> PID_thrust/1
  Subsystem/1(x) -> Scope6/1  "x"
  Mux/1 -> [Reference]
  Subsystem/3(z) -> Scope6/3  "z"
  PID_roll/1 -> Motors command calculation/2(roll_cmd), Scope8/1
  Demux3/3 -> Subsystem/3(z(t)), Bus Creator2/3  "z(t)"
  Bus Selector/1 -> Sum3/2  "<z(t)>"
  Sum4/1 -> PID_pitch/1
  World to Body/2(y_ref_) -> Sum2/1, Mux/2
  Subsystem1/1(e_norm) -> PID_yaw/1
  Bus Selector1/2 -> Sum4/2  "<pitch>"
  Degrees to Radians/1 -> Sum6/1
  PID_pitch_desired/1 -> Gain/1
  [Reference] -> Subsystem/4(In2), Subsystem2/4(In1)
  Clock/1 -> MATLAB Function1/1(sim_time)
  Demux4/1 -> Subsystem2/1(roll), Bus Creator1/1  "roll"
  PID_pitch/1 -> Gain1/1
  Saturation/1 -> Motors command calculation/1(thrust_cmd), Scope1/1
  Manual Switch1/1 -> Mux/6, Degrees to Radians/1  "yaw_{ref} [deg]"
  Demux3/2 -> Subsystem/2(y(t)), Bus Creator2/2  "y(t)"
  Demux4/2 -> Subsystem2/2(pitch), Bus Creator1/2  "pitch"
  Sum1/1 -> PID_roll/1
  Sum5/1 -> PID_pitch_desired/1  "x_ref"
  Demux4/3 -> Subsystem2/3(yaw), Bus Creator1/3  "yaw"
  Bus Selector/2 -> Sum5/2  "<x(t)>"
  Subsystem/2(y) -> Scope6/2  "y"
  World to Body/1(x_ref_) -> Sum5/1, Mux/1
  Sum6/1 -> Subsystem1/1(e)
  Bus Selector1/3 -> Sum6/2  "<yaw>"
  Bus Selector1/1 -> Sum1/2  "<roll>"
  Bus Creator1/1 -> Bus Selector1/1
  Bus Creator2/1 -> Bus Selector/1
  Manual Switch2/1 -> Sum3/1, Mux/3  "z_{ref} [m]"
  DronPos/1 -> Demux3/1  "[x;y;z]"
  Mux6/1 -> Demux4/1  "[roll;pitch;yaw] [rad]"
  Mux7/1 -> Radians to Degrees3/1  "[alpha;beta] [rad]"
  otacky^2 na sily/1(u) -> Demux/1  "[T; moments]"
  Radians to Degrees3/1 -> Scope2/1  "[a;b] [deg]"
  Demux/1 -> Scope/1  "T"
  Demux/2 -> Mux1/1
  Demux/3 -> Mux1/2
  Demux/4 -> Mux1/3
  Mux1/1 -> Scope/2  "moments"
  Max rotation^2/1 -> To Workspace/1, otacky^2 na sily/1(U), Scope10/1
  Radians to Degrees4/1 -> Scope7/2, Mux/4
  PID_thrust/1 -> Saturation/1
  PID_roll_desired/1 -> Sum1/1, Radians to Degrees4/1  "roll_ref"
  Constant6/1 -> World to Body/2(y_ref)  "y_{ref}"
  Gain/1 -> Radians to Degrees5/1, Sum4/1  "pitch_ref"
  Radians to Degrees5/1 -> Scope7/1, Mux/5
  Manual Switch/1 -> World to Body/1(x_ref)  "x_{ref} [m]"
  Motors command calculation/1(U1) -> Mux12/1
  Motors command calculation/3(U3) -> Mux12/3
  Motors command calculation/2(U2) -> Mux12/2
  Motors command calculation/4(U4) -> Mux12/4
  Mux12/1 -> Max rotation^2/1
  DronRotM/1 -> Uhly koptery [rad]/1(RotM)
  PendPos/1 -> Scope9/1  "x y z zavazi"
  Uhly koptery [rad]/2(pitch) -> Mux6/2
  Uhly zavazi [rad]/2(beta_rad) -> Mux7/2
  Uhly koptery [rad]/3(yaw) -> Mux6/3
  PendRotM/1 -> Uhly zavazi [rad]/1(RotM)
  Uhly koptery [rad]/1(roll) -> Mux6/1
  Uhly zavazi [rad]/1(alpha_rad) -> Mux7/1
  Subsystem2/1(Out1) -> Scope5/1  "roll"
  Subsystem2/2(Out2) -> Scope5/2  "pitch"
  Subsystem2/3(Out3) -> Scope5/3  "yaw"
  time/1 -> Scope4/1
  Step/1 -> Manual Switch/2
  Constant5/1 -> Manual Switch/1
  Constant1/1 -> Manual Switch1/1
  Step1/1 -> Manual Switch1/2
  Constant2/1 -> Manual Switch2/1
  Step2/1 -> Manual Switch2/2
  Gain1/1 -> Scope18/1, Motors command calculation/3(pitch_cmd)

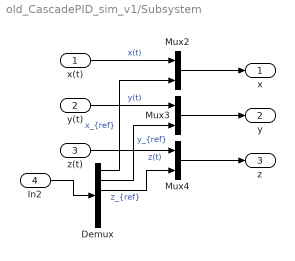
== system old_CascadePID_sim_v1/Subsystem ==
  x(t) : Inport
  y(t) : Inport  Port=2
  z(t) : Inport  Port=3
  In2 : Inport  Port=4
  Demux : Demux  Outputs=6
  Mux2 : Mux  Inputs=2
  Mux3 : Mux  Inputs=2
  Mux4 : Mux  Inputs=2
  x : Outport
  y : Outport  Port=2
  z : Outport  Port=3
  wires:
  Demux/2 -> Mux3/2  "y_{ref}"
  Mux4/1 -> z/1
  y(t)/1 -> Mux3/1  "y(t)"
  Mux3/1 -> y/1
  Demux/1 -> Mux2/2  "x_{ref}"
  Demux/3 -> Mux4/2  "z_{ref}"
  Mux2/1 -> x/1
  In2/1 -> Demux/1
  x(t)/1 -> Mux2/1  "x(t)"
  z(t)/1 -> Mux4/1  "z(t)"

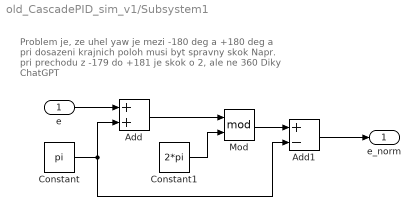
== system old_CascadePID_sim_v1/Subsystem1 ==
  note: Problem je, ze uhel yaw je mezi -180 deg a +180 deg
      | a pri dosazeni krajnich poloh musi byt spravny skok
      | Napr. pri prechodu z -179 do +181 je skok o 2, ale ne 360
      | Diky ChatGPT
  e : Inport
  Add : Sum
  Add1 : Sum  Inputs=+-
  Constant : Constant  Value=pi
  Constant1 : Constant  Value=2*pi
  Mod : Math  Operator=mod
  e_norm : Outport
  wires:
  e/1 -> Add/1
  Add/1 -> Mod/1
  Constant/1 -> Add1/2, Add/2
  Constant1/1 -> Mod/2
  Mod/1 -> Add1/1
  Add1/1 -> e_norm/1

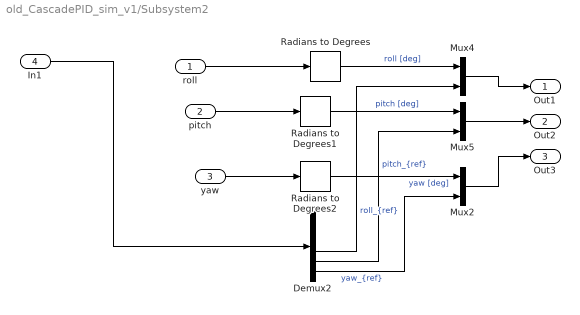
== system old_CascadePID_sim_v1/Subsystem2 ==
  roll : Inport
  pitch : Inport  Port=2
  yaw : Inport  Port=3
  In1 : Inport  Port=4
  Demux2 : Demux  Outputs=6
  Mux2 : Mux  Inputs=2
  Mux4 : Mux  Inputs=2
  Mux5 : Mux  Inputs=2
  Radians to Degrees : simulink_extras/Transformations/Radians to Degrees
  Radians to Degrees1 : simulink_extras/Transformations/Radians to Degrees
  Radians to Degrees2 : simulink_extras/Transformations/Radians to Degrees
  Out1 : Outport
  Out2 : Outport  Port=2
  Out3 : Outport  Port=3
  wires:
  Radians to Degrees/1 -> Mux4/1  "roll [deg]"
  Demux2/6 -> Mux2/2  "yaw_{ref}"
  Demux2/5 -> Mux5/2  "pitch_{ref}"
  Radians to Degrees1/1 -> Mux5/1  "pitch [deg]"
  Demux2/4 -> Mux4/2  "roll_{ref}"
  Radians to Degrees2/1 -> Mux2/1  "yaw [deg]"
  roll/1 -> Radians to Degrees/1
  yaw/1 -> Radians to Degrees2/1
  pitch/1 -> Radians to Degrees1/1
  Mux5/1 -> Out2/1
  In1/1 -> Demux2/1
  Mux4/1 -> Out1/1
  Mux2/1 -> Out3/1

== matlab function old_CascadePID_sim_v1/Uhly koptery [rad] ==
  data: RotM input; roll output; pitch output; yaw output
function [roll, pitch, yaw] = quad_attitude(RotM)
% matice rotace koptery z Python, vuci svetu!!!
% rotm2eul prevadi na Eulerove uhly
radians = rotm2eul(RotM, 'ZYX'); % pouzivam poradi ZYX

% roll = kolem x, pitch = kolem y, yaw = kolem z
yaw = radians(1);
pitch = radians(2);
roll = radians(3);
end

== matlab function old_CascadePID_sim_v1/MATLAB Function1 ==
  data: x_ref output; y_ref output; z_ref output; sim_time input; yaw_ref output
function [x_ref, y_ref, z_ref, yaw_ref] = fcn(sim_time)
if sim_time < 10
    z_ref = 8;
    x_ref = 0;
    y_ref = 0;
    yaw_ref = 0;
elseif sim_time < 20
    z_ref = 15;
    x_ref = 10;
    y_ref = 0;
    yaw_ref = 45;
elseif sim_time < 25
    z_ref = 8;
    x_ref = 10;
    y_ref = -5;
    yaw_ref = -45;
elseif sim_time < 30
    z_ref = 10;
    x_ref = -5;
    y_ref = -10;
    yaw_ref = -15;
elseif sim_time < 40
    z_ref = 12;
    x_ref = -5;
    y_ref = 0;
    yaw_ref = 30;
else
    x_ref = 0; % [m]
    y_ref = 0; % [m]
    z_ref = 10; % [m]
    yaw_ref = 0; %[deg] mezi -180 deg a +180 deg
end

== matlab function old_CascadePID_sim_v1/Motors command calculation ==
  data: thrust_cmd input; U1 output; roll_cmd input; pitch_cmd input; yaw_cmd input; U2 output; U3 output; U4 output
function [U1, U2, U3, U4] = fcn(thrust_cmd, roll_cmd, pitch_cmd, yaw_cmd)

U1 = thrust_cmd+roll_cmd-pitch_cmd+yaw_cmd;
U2 = thrust_cmd-roll_cmd-pitch_cmd-yaw_cmd;
U3 = thrust_cmd-roll_cmd+pitch_cmd+yaw_cmd;
U4 = thrust_cmd+roll_cmd+pitch_cmd-yaw_cmd;

== matlab function old_CascadePID_sim_v1/World to Body ==
  data: x_ref input; x_ref_ output; y_ref input; yaw input; y_ref_ output
function [x_ref_, y_ref_]= fcn(x_ref, y_ref, yaw)
R_z = [cos(yaw), -sin(yaw), 0; 
       sin(yaw), cos(yaw), 0; 
       0, 0, 1];

out = R_z\[x_ref; y_ref; 0];
%out = [x_ref, y_ref];
x_ref_ = out(1);
y_ref_ = out(2);

== matlab function old_CascadePID_sim_v1/otacky^2 na sily ==
  data: u output; U input; k_thrust parameter; b_moment parameter; l parameter
function u = fcn(U, k_thrust, b_moment, l)
U1 = U(1);
U2 = U(2);
U3 = U(3);
U4 = U(4);

T = k_thrust*(U1+U2+U3+U4);
Tau_roll = k_thrust*l*(U1+U4-U2-U3);
Tau_pitch = k_thrust*l*(U3+U4-U1-U2);
Tau_yaw = b_moment*(U1+U3-U2-U4);

u = [T; Tau_roll; Tau_pitch; Tau_yaw]; %[tahova sila; momenty]

== matlab function old_CascadePID_sim_v1/Uhly zavazi [rad] ==
  data: RotM input; alpha_rad output; beta_rad output
function [alpha_rad, beta_rad] = pend_orient(RotM)
% Расчет углов альфа и бета маятника

% Вектор маятника
rope_vector = RotM * [0; 0; -1];

% Расчет угла альфа
rope_vector_xz = rope_vector([1, 3]); % Компоненты x и z
z_axis = [0; -1];
cos_alpha = dot(rope_vector_xz, z_axis) / (norm(rope_vector_xz) * norm(z_axis));
cos_alpha = max(-1, min(1, cos_alpha)); % Ограничиваем в диапазоне [-1, 1]
alpha = acos(cos_alpha);
if rope_vector(1) < 0
    alpha = -alpha;
end

% Расчет угла бета
rope_vector_xz_3 = [rope_vector(1); 0; rope_vector(3)];
cos_beta = dot(rope_vector, rope_vector_xz_3) / (norm(rope_vector) * norm(rope_vector_xz_3));
cos_beta = max(-1, min(1, cos_beta)); % Ограничиваем в диапазоне [-1, 1]
beta = acos(cos_beta);
if rope_vector(2) < 0
    beta = -beta;
end

% Округляем до 5 знаков после запятой
% alpha_rad = round(alpha, 5); %[rad]
% beta_rad = round(beta, 5); %[rad]
alpha_rad = alpha;
beta_rad = beta;
